simulink model "Transformada_directa_Park"  (R2023b)
settings: Solver=ode4  StartTime=0.0  StopTime=10.0  FixedStep=1e-5  RelTol=1e-3
settings Model: Creator=Julya  LastModifiedBy=Julya

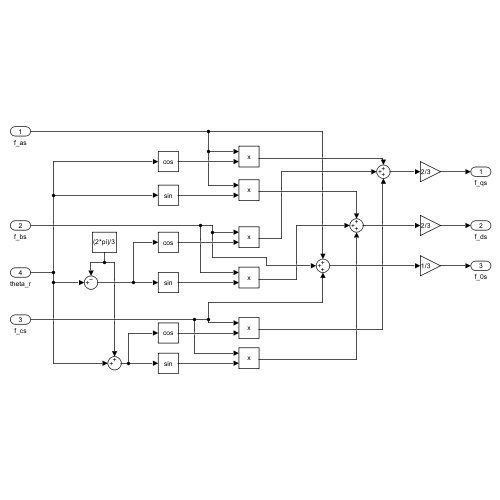
[thumbnail: Simulink's stored preview of the top-level diagram]
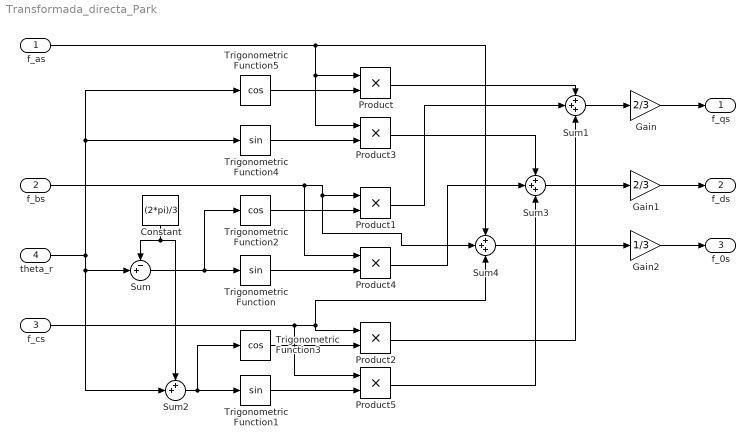
== system Transformada_directa_Park ==
  f_as : Inport
  f_bs : Inport  Port=2
  f_cs : Inport  Port=3
  theta_r : Inport  Port=4
  Constant : Constant  Value=(2*pi)/3
  Gain : Gain  Gain=2/3
  Gain1 : Gain  Gain=2/3
  Gain2 : Gain  Gain=1/3
  Product{,1..5} (6 alike) : Product
  Sum : Sum  Inputs=-+|
  Sum1 : Sum  Inputs=+++
  Sum2 : Sum  Inputs=++|
  Sum3 : Sum  Inputs=+++
  Sum4 : Sum  Inputs=+++
  Trigonometric Function : Trigonometry
  Trigonometric Function1 : Trigonometry
  Trigonometric Function2 : Trigonometry  Operator=cos
  Trigonometric Function3 : Trigonometry  Operator=cos
  Trigonometric Function4 : Trigonometry
  Trigonometric Function5 : Trigonometry  Operator=cos
  f_qs : Outport
  f_ds : Outport  Port=2
  f_0s : Outport  Port=3
  wires:
  theta_r/1 -> Sum2/2, Sum/2, Trigonometric Function5/1, Trigonometric Function4/1
  Constant/1 -> Sum/1, Sum2/1
  Sum/1 -> Trigonometric Function/1, Trigonometric Function2/1
  Sum2/1 -> Trigonometric Function3/1, Trigonometric Function1/1
  f_as/1 -> Sum4/1, Product3/1, Product/1
  Trigonometric Function5/1 -> Product/2
  Product/1 -> Sum1/1
  Trigonometric Function2/1 -> Product1/2
  f_bs/1 -> Sum4/2, Product1/1, Product4/1
  Product1/1 -> Sum1/2
  Trigonometric Function3/1 -> Product2/2
  f_cs/1 -> Sum4/3, Product2/1, Product5/1
  Product2/1 -> Sum1/3
  Sum1/1 -> Gain/1
  Gain/1 -> f_qs/1
  Trigonometric Function4/1 -> Product3/2
  Trigonometric Function/1 -> Product4/2
  Trigonometric Function1/1 -> Product5/2
  Product3/1 -> Sum3/1
  Product4/1 -> Sum3/2
  Product5/1 -> Sum3/3
  Sum3/1 -> Gain1/1
  Gain1/1 -> f_ds/1
  Sum4/1 -> Gain2/1
  Gain2/1 -> f_0s/1
